simulink model "Week2_Problem4"  (R2020a)
settings: Solver=ode15s  StartTime=0.0  StopTime=0.4  RelTol=1e-3
values from neighbouring files (symbols this model uses):
  b = 3.5077E-6    [ModelData.sldd]    (also in ModelData1.sldd)
  D = 0.0    [ModelData1.sldd]
  I = 1.0    [ModelData1.sldd]
  J = 3.2284E-6    [ModelData.sldd]    (also in ModelData1.sldd)
  K = 0.0274    [ModelData.sldd]    (also in ModelData1.sldd)
  L = 2.75E-6    [ModelData.sldd]    (also in ModelData1.sldd)
  P = 1.0    [ModelData1.sldd]
  R = 4.0    [ModelData.sldd]    (also in ModelData1.sldd)
settings Model: DataDictionary=ModelData1.sldd  Creator=tnradm  LastModifiedBy=tnradm

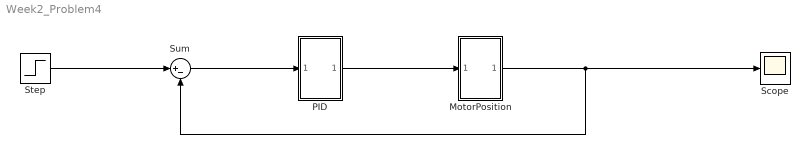
== system Week2_Problem4 ==
  MotorPosition : Subsystem
  PID : Subsystem
  Scope : Scope
  Step : Step  Time=0  SampleTime=0
  Sum : Sum  Inputs=|+-
  wires:
  MotorPosition/1(Out1) -> Sum/2, Scope/1
  Sum/1 -> PID/1(In1)
  Step/1 -> Sum/1
  PID/1(Out1) -> MotorPosition/1(In1)

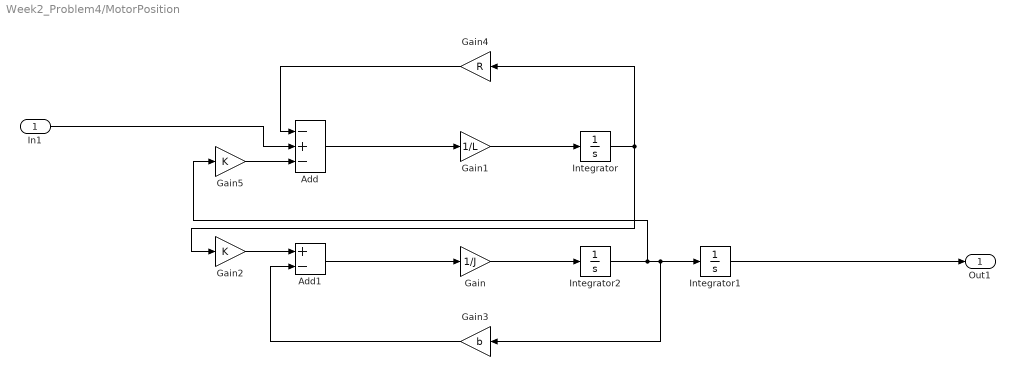
== system Week2_Problem4/MotorPosition ==
  In1 : Inport
  Add : Sum  Inputs=-+-
  Add1 : Sum  Inputs=+-
  Gain : Gain  Gain=1/J
  Gain1 : Gain  Gain=1/L
  Gain2 : Gain  Gain=K
  Gain3 : Gain  Gain=b
  Gain4 : Gain  Gain=R
  Gain5 : Gain  Gain=K
  Integrator : Integrator
  Integrator1 : Integrator
  Integrator2 : Integrator
  Out1 : Outport
  wires:
  Gain2/1 -> Add1/1
  Gain5/1 -> Add/3
  Add/1 -> Gain1/1
  Integrator/1 -> Gain2/1, Gain4/1
  Gain3/1 -> Add1/2
  Integrator1/1 -> Out1/1
  Integrator2/1 -> Gain5/1, Gain3/1, Integrator1/1
  Add1/1 -> Gain/1
  Gain4/1 -> Add/1
  Gain1/1 -> Integrator/1
  Gain/1 -> Integrator2/1
  In1/1 -> Add/2

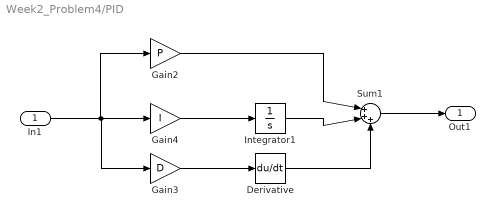
== system Week2_Problem4/PID ==
  In1 : Inport
  Derivative : Derivative
  Gain2 : Gain  Gain=P
  Gain3 : Gain  Gain=D
  Gain4 : Gain  Gain=I
  Integrator1 : Integrator
  Sum1 : Sum  Inputs=|+++
  Out1 : Outport
  wires:
  In1/1 -> Gain2/1, Gain4/1, Gain3/1
  Integrator1/1 -> Sum1/2
  Derivative/1 -> Sum1/3
  Gain3/1 -> Derivative/1
  Sum1/1 -> Out1/1
  Gain2/1 -> Sum1/1
  Gain4/1 -> Integrator1/1
